simulink model "lc_filt_2"  (Simulink 7.4)
settings: Solver=ode45  StartTime=0.0  StopTime=10.0  MaxStep=1/(5*5e6)  RelTol=1e-3
InitFcn:
  | [l,c]=qsynth('getLC')
values from neighbouring files (symbols this model uses):
  a = [1 5726176.52661 1.28574552517e+14 5.97941269361e+20 5.92183808786e+27 2.12384980348e+34 1.13676377206e+41 2.81047410932e+47 7.39377027116e+53 8.72797204109e+59]    [lpf_coefs.mat]    (also in qsynth.m = 1)
  b = [0 36915.6508509 -1.25549596846e-06 1.20108825102e+19 -347373112.51 1.28132141519e+33 -2.666806229e+22 5.6099849733e+46 -6.09794797058e+35 8.72797204109e+59]    [lpf_coefs.mat]    (also in qsynth.m = 0)
  c = [1.7464e-07 0 2.8303e-07 0 2.0989e-07 0 1.304e-07 0 4.9154e-08]    [lcvalues.mat]    (also in qsynth.m = 1/val1)
  d = 1    [qsynth.m]
  l = [0 2.1751e-07 2.1186e-08 2.0002e-07 7.2973e-08 1.4884e-07 1.5754e-07 1.3878e-07 4.5617e-07]    [lcvalues.mat]
undefined symbols (not defined in the file or in its folder): Fs, magnitude
libraries: powerlib x14, dspindex x6, dspsigops x3, dspbuff3 x2, dspxfrm3 x2, dsparch3 x2, dspsnks4 x2, dspmtrx3 x1, simulink x1
settings Model: Creator=Owner  LastModifiedBy=Dick
settings DataIOCC: SignalLoggingName=sigsOut
settings OptimizationCC: BooleanDataType=off  InlineInvariantSignals=on  InitFltsAndDblsToZero=on
settings DebuggingCC: SaveWithParameterizedLinksMsg=none  SignalResolutionControl=TryResolveAllWithWarning  SolverPrmCheckMsg=none  MultiTaskDSMMsg=warning  MultiTaskCondExecSysMsg=none  StrictBusMsg=None
settings HardwareCC: TargetUnknown=on
settings RTWCC: IncludeERTFirstTime=on
settings GRTTargetCC: TargetFcnLib=ansi_tfl_tmw.mat

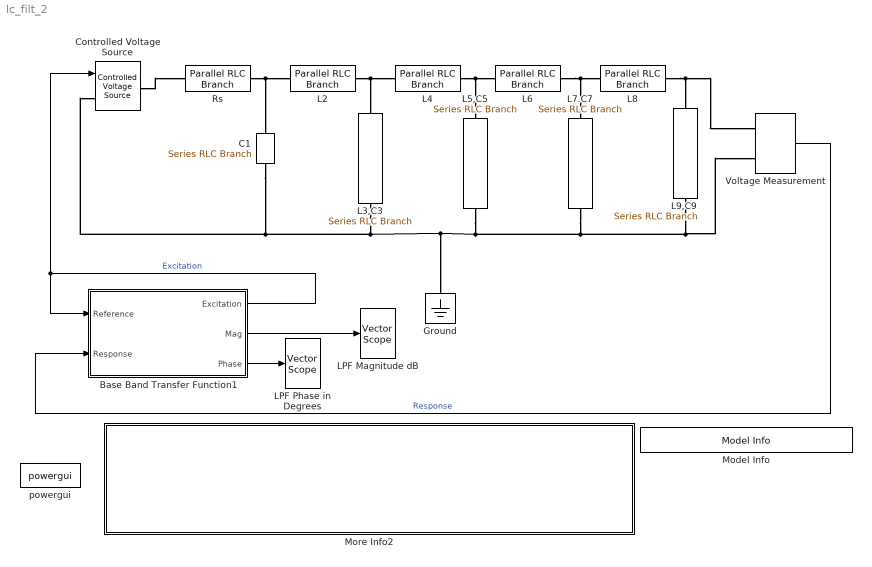
== system lc_filt_2 ==
  " L2" : powerlib/Elements/Parallel RLC Branch  DialogController=POWERSYS.PowerSysDialog  PhysicalDomain=powersysdomain  SubClassName=unknown  LeftPortType=p1  RightPortType=p1  LConnTagsString=a  RConnTagsString=__new0  BranchType=L  Resistance=1.0  Inductance=l(2)  SetiL0=off  InitialCurrent=0  Capacitance=1.0  Setx0=off  InitialVoltage=0  Measurements=None
  " L4" : powerlib/Elements/Parallel RLC Branch  DialogController=POWERSYS.PowerSysDialog  PhysicalDomain=powersysdomain  SubClassName=unknown  LeftPortType=p1  RightPortType=p1  LConnTagsString=a  RConnTagsString=__new0  BranchType=L  Resistance=1.0  Inductance=l(4)  SetiL0=off  InitialCurrent=0  Capacitance=1.0  Setx0=off  InitialVoltage=0  Measurements=None
  " L6" : powerlib/Elements/Parallel RLC Branch  DialogController=POWERSYS.PowerSysDialog  PhysicalDomain=powersysdomain  SubClassName=unknown  LeftPortType=p1  RightPortType=p1  LConnTagsString=a  RConnTagsString=__new0  BranchType=L  Resistance=1.0  Inductance=l(6)  SetiL0=off  InitialCurrent=0  Capacitance=1.0  Setx0=off  InitialVoltage=0  Measurements=None
  " L8" : powerlib/Elements/Parallel RLC Branch  DialogController=POWERSYS.PowerSysDialog  PhysicalDomain=powersysdomain  SubClassName=unknown  LeftPortType=p1  RightPortType=p1  LConnTagsString=a  RConnTagsString=__new0  BranchType=L  Resistance=1.0  Inductance=l(8)  SetiL0=off  InitialCurrent=0  Capacitance=1.0  Setx0=off  InitialVoltage=0  Measurements=None
  " Rs" : powerlib/Elements/Parallel RLC Branch  DialogController=POWERSYS.PowerSysDialog  PhysicalDomain=powersysdomain  SubClassName=unknown  LeftPortType=p1  RightPortType=p1  LConnTagsString=a  RConnTagsString=__new0  BranchType=R  Resistance=1  Inductance=1.0  SetiL0=off  InitialCurrent=0  Capacitance=1.0  Setx0=off  InitialVoltage=0  Measurements=None
  Base Band Transfer Function1 : Subsystem  Description=Spectrum Analyzer  mask{BW=5e6, NFFT=1024, Avg_fac=100}
      mask prompts: BW "Bandwidth"; NFFT "FFT Length (power of 2)"; Avg_fac "Averaging Factor (>=1)"
  C1 : powerlib/Elements/Series RLC Branch  DialogController=POWERSYS.PowerSysDialog  PhysicalDomain=powersysdomain  SubClassName=unknown  LeftPortType=p1  RightPortType=p1  LConnTagsString=__new0  RConnTagsString=__new0  BranchType=C  Resistance=1.0  Inductance=1.0  SetiL0=off  InitialCurrent=0  Capacitance=c(1)  Setx0=off  InitialVoltage=0  Measurements=None
  Controlled Voltage Source : powerlib/Electrical Sources/Controlled Voltage Source  DialogController=POWERSYS.PowerSysDialog  SystemSampleTime=-1  Initialize=off  Source_Type=AC  Amplitude=100  Phase=0  Frequency=0  Measurements=Voltage
  Ground : powerlib/Elements/Ground  DialogController=POWERSYS.PowerSysDialog  PhysicalDomain=powersysdomain  SubClassName=unknown  LeftPortType=p1  RightPortType=p1  LConnTagsString=a
  L3,C3 : powerlib/Elements/Series RLC Branch  DialogController=POWERSYS.PowerSysDialog  PhysicalDomain=powersysdomain  SubClassName=unknown  LeftPortType=p1  RightPortType=p1  LConnTagsString=__new0  RConnTagsString=__new0  BranchType=LC  Resistance=1.0  Inductance=l(3)  SetiL0=off  InitialCurrent=0  Capacitance=c(3)  Setx0=off  InitialVoltage=0  Measurements=None
  L5,C5 : powerlib/Elements/Series RLC Branch  DialogController=POWERSYS.PowerSysDialog  PhysicalDomain=powersysdomain  SubClassName=unknown  LeftPortType=p1  RightPortType=p1  LConnTagsString=__new0  RConnTagsString=__new0  BranchType=LC  Resistance=1.0  Inductance=l(5)  SetiL0=off  InitialCurrent=0  Capacitance=c(5)  Setx0=off  InitialVoltage=0  Measurements=None
  L7.C7 : powerlib/Elements/Series RLC Branch  DialogController=POWERSYS.PowerSysDialog  PhysicalDomain=powersysdomain  SubClassName=unknown  LeftPortType=p1  RightPortType=p1  LConnTagsString=__new0  RConnTagsString=__new0  BranchType=LC  Resistance=1.0  Inductance=l(7)  SetiL0=off  InitialCurrent=0  Capacitance=c(7)  Setx0=off  InitialVoltage=0  Measurements=None
  "L9,C9 " : powerlib/Elements/Series RLC Branch  DialogController=POWERSYS.PowerSysDialog  PhysicalDomain=powersysdomain  SubClassName=unknown  LeftPortType=p1  RightPortType=p1  LConnTagsString=__new0  RConnTagsString=__new0  BranchType=LC  Resistance=1.0  Inductance=l(9)  SetiL0=off  InitialCurrent=0  Capacitance=c(9)  Setx0=off  InitialVoltage=0  Measurements=None
  LPF Magnitude dB : dspsnks4/Vector Scope  DialogController=dspdialog.VectorScope  DialogControllerArgs=DataTag5  ScopeProperties=on  Domain=Frequency  HorizSpan=1  DisplayProperties=off  AxisGrid=on  Memory=off  FrameNumber=on  AxisLegend=off  AxisZoom=off  OpenScopeAtSimStart=on  OpenScopeImmediately=off  FigPos=[15 321 372 236]  AxisProperties=off  XUnits=Hertz  XRange=[0...Fs/2]  InheritXIncr=on  XIncr=2*Fs  XLabel=Time  XLimit=Auto  XMin=0  XMax=1  XStart=0  YUnits=dB  YLabel=dB  LineProperties=off  LineColors=[1 0 0]|[1 0 0]  XAxisParamsVer=6.8
      settings: YMin=-100  YMax=10
  LPF Phase in Degrees : dspsnks4/Vector Scope  DialogController=dspdialog.VectorScope  DialogControllerArgs=DataTag6  ScopeProperties=on  Domain=Frequency  HorizSpan=1  DisplayProperties=off  AxisGrid=on  Memory=off  FrameNumber=on  AxisLegend=off  AxisZoom=off  OpenScopeAtSimStart=on  OpenScopeImmediately=off  FigPos=[16 37 372 236]  AxisProperties=off  XUnits=Hertz  XRange=[0...Fs/2]  InheritXIncr=on  XIncr=1  XLabel=Frequency  XLimit=Auto  XMin=0  XMax=1  XStart=0  YUnits=Magnitude  YLabel=Phase in Degrees  LineProperties=off  LineColors=[1 0 0]  XAxisParamsVer=6.8
      settings: YMin=-892.290290597093  YMax=45.3005092441757
  Model Info : simulink/Model-Wide Utilities/Model Info  SystemSampleTime=-1  InitialBlockCM=None  BlockCM=None  Frame=on  DisplayStringWithTags=Copywrite 2005-2010 The MathWorks, Inc.  HorizontalTextAlignment=Center  LeftAlignmentValue=0.5  SourceBlockDiagram=lc_filt_2  TagMaxNumber=20
  More Info2 : Subsystem
      settings: OpenFcn=qsynth
      mask Display: disp('1) Double click here to synthesize LC filter. Use N=9, Rs=1 Rl=inf Fc=1e6 \n 2) Synthesize the filter, do not close GUI,  then return to this model and start the simulation. \n 3) The LC filter is "measured" with the Base Band Transfer Function Estimator \n ')
  Voltage Measurement : powerlib/Measurements/Voltage Measurement  DialogController=POWERSYS.PowerSysDialog  SystemSampleTime=-1  PhasorSimulation=off  OutputType=Magnitude  PSBequivalent=0
  powergui : powerlib/powergui  SystemSampleTime=-1  SimulationMode=Continuous  SampleTime=0  frequency=60  SPID=off  DisableSnubberDevices=off  DisableRonSwitches=off  DisableVfSwitches=off  SwTol=0  Interpol=off  frequencyindice=0  echomessages=off  HookPort=off  DisplayEquations=off  FunctionMessages=off  EnableUseOfTLC=off  x0status=blocks  RestoreLinks=warning  Frange=[0:2:500]  Ylog=off  Xlog=on  ShowGrid=off  save=off  variable=ZData  ZoomFFT=on  StartTime=0.0  cycles=1  DisplayStyle=1  fundamental=60  FreqAxis=off  MaxFrequency=1000  frequencyindicesteady=1  RmsSteady=1  display=off  Ts=0  methode=off
  wires:
  Voltage Measurement/1 -> Base Band Transfer Function1/2(Response)  "Response"
  Base Band Transfer Function1/2(Mag) -> LPF Magnitude dB/1
  Base Band Transfer Function1/3(Phase) -> LPF Phase in Degrees/1
  Base Band Transfer Function1/1(Excitation) -> Controlled Voltage Source/1, Base Band Transfer Function1/1("Reference ")  "Excitation"
  connections:
  " Rs"/RConn1 -- C1/LConn1 -- " L2"/LConn1
  " L2"/RConn1 -- L3,C3/LConn1 -- " L4"/LConn1
  " L4"/RConn1 -- L5,C5/LConn1 -- " L6"/LConn1
  " L6"/RConn1 -- L7.C7/LConn1 -- " L8"/LConn1
  L5,C5/RConn1 -- L7.C7/RConn1 -- "L9,C9 "/RConn1 -- Voltage Measurement/LConn2 -- L3,C3/RConn1 -- C1/RConn1 -- Controlled Voltage Source/LConn1 -- Ground/LConn1
  Controlled Voltage Source/RConn1 -- " Rs"/LConn1
  " L8"/RConn1 -- Voltage Measurement/LConn1 -- "L9,C9 "/LConn1

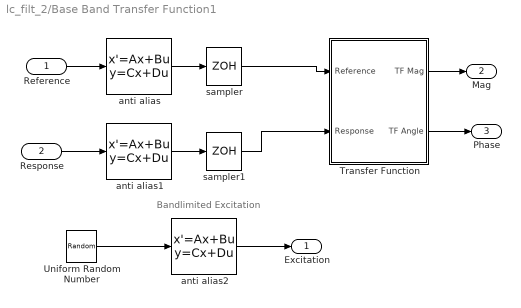
== system lc_filt_2/Base Band Transfer Function1 ==
  note: Bandlimited Excitation
  "Reference " : Inport  OutDataType=sfix(16)  OutScaling=2^0
  Response : Inport  Port=2  OutDataType=sfix(16)  OutScaling=2^0
  "Transfer Function " : Subsystem  mask{NFFT=NFFT, Navg=Avg_fac, pcnt=100/1.28, unwrap_flag=on}
      mask prompts: NFFT "FFT length (power of 2):"; Navg "Spectral Averaging Factor (>=1):"; pcnt "Percentage of  Alias Free Data  (<=100)"; unwrap_flag "Unwrap Phase"
      mask Display: disp('Transfer Function \n Estimation (v2.0) ')
  Uniform Random Number : UniformRandomNumber  SampleTime=1/(2.56*BW)
  anti alias : StateSpace  AncestorBlock=dsparch3/Analog Filter Design  A=a  B=b  C=c  D=d  mask(Analog Filter Design){method=Elliptic, filttype=Lowpass, N=8, Wlo=BW*2*pi, Whi=80, Rp=2, Rs=100}
      mask prompts: method "Design method:"; filttype "Filter type:"; N "Filter order:"; Wlo "Passband edge frequency (rad/s):"; Whi "(unused)"; Rp "Passband ripple in dB:"; Rs "Stopband attenuation in dB:"
      mask help: Design one of several standard analog filters, implemented in state-space form.
      mask init:
      | [a,b,c,d,h,w,str]=dspblkanalog('design', method,filttype,N,Wlo,Whi,Rp,Rs);
      mask Help: web(dspbhelp);
      mask StyleString: popup(Butterworth|Chebyshev I|Chebyshev II|Elliptic|Bessel),popup(Lowpass|Highpass|Bandpass|Bandstop),edit,edit,edit,edit,edit
      mask CallbackString: dspblkanalog|dspblkanalog|||||
      mask Display: plot(w,h); text(.05,.9,str);
  anti alias1 : StateSpace  AncestorBlock=dsparch3/Analog Filter Design  A=a  B=b  C=c  D=d  mask(Analog Filter Design){method=Elliptic, filttype=Lowpass, N=8, Wlo=BW*2*pi, Whi=80, Rp=2, Rs=100}
      mask prompts: method "Design method:"; filttype "Filter type:"; N "Filter order:"; Wlo "Passband edge frequency (rad/s):"; Whi "(unused)"; Rp "Passband ripple in dB:"; Rs "Stopband attenuation in dB:"
      mask help: Design one of several standard analog filters, implemented in state-space form.
      mask init:
      | [a,b,c,d,h,w,str]=dspblkanalog('design', method,filttype,N,Wlo,Whi,Rp,Rs);
      mask Help: web(dspbhelp);
      mask StyleString: popup(Butterworth|Chebyshev I|Chebyshev II|Elliptic|Bessel),popup(Lowpass|Highpass|Bandpass|Bandstop),edit,edit,edit,edit,edit
      mask CallbackString: dspblkanalog|dspblkanalog|||||
      mask Display: plot(w,h); text(.05,.9,str);
  anti alias2 : StateSpace  AncestorBlock=dsparch3/Analog Filter Design  A=a  B=b  C=c  D=d  mask(Analog Filter Design){method=Elliptic, filttype=Lowpass, N=8, Wlo=BW*2*pi, Whi=80, Rp=2, Rs=100}
      mask prompts: method "Design method:"; filttype "Filter type:"; N "Filter order:"; Wlo "Passband edge frequency (rad/s):"; Whi "(unused)"; Rp "Passband ripple in dB:"; Rs "Stopband attenuation in dB:"
      mask help: Design one of several standard analog filters, implemented in state-space form.
      mask init:
      | [a,b,c,d,h,w,str]=dspblkanalog('design', method,filttype,N,Wlo,Whi,Rp,Rs);
      mask Help: web(dspbhelp);
      mask StyleString: popup(Butterworth|Chebyshev I|Chebyshev II|Elliptic|Bessel),popup(Lowpass|Highpass|Bandpass|Bandstop),edit,edit,edit,edit,edit
      mask CallbackString: dspblkanalog|dspblkanalog|||||
      mask Display: plot(w,h); text(.05,.9,str);
  sampler : ZeroOrderHold  SampleTime=1/(2.56*BW)
  sampler1 : ZeroOrderHold  SampleTime=1/(2.56*BW)
  Excitation : Outport  OutDataType=sfix(16)  OutScaling=2^0
  Mag : Outport  Port=2  OutDataType=sfix(16)  OutScaling=2^0
  Phase : Outport  Port=3  OutDataType=sfix(16)  OutScaling=2^0
  wires:
  "Transfer Function "/2(TF Angle) -> Phase/1
  "Transfer Function "/1(TF Mag) -> Mag/1
  sampler1/1 -> "Transfer Function "/2(Response)
  sampler/1 -> "Transfer Function "/1(Reference)
  anti alias2/1 -> Excitation/1
  Uniform Random Number/1 -> anti alias2/1
  Response/1 -> anti alias1/1
  anti alias1/1 -> sampler1/1
  "Reference "/1 -> anti alias/1
  anti alias/1 -> sampler/1

== system lc_filt_2/More Info2 ==

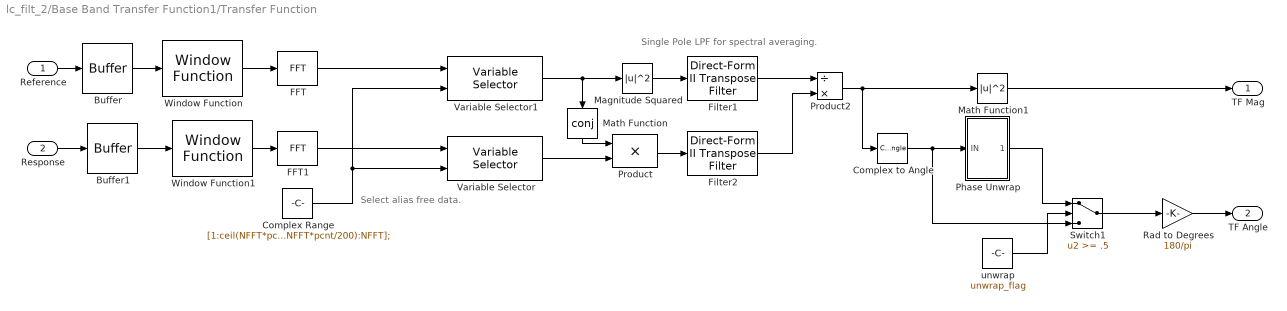
== system lc_filt_2/Base Band Transfer Function1/Transfer Function  ==
  note: Single Pole LPF for spectral averaging.
  note: Select alias free data.
  Reference : Inport  OutDataType=sfix(16)  OutScaling=2^0
  Response : Inport  Port=2  OutDataType=sfix(16)  OutScaling=2^0
  Buffer : dspbuff3/Buffer  N=NFFT  V=0  ic=0
  Buffer1 : dspbuff3/Buffer  N=NFFT  V=0  ic=0
  Complex Range : Constant  Value=[1:ceil(NFFT*pcnt/200),ceil(1+NFFT-NFFT*pcnt/200):NFFT];  OutDataType=sfix(16)  OutScaling=2^0
  Complex to Angle : ComplexToMagnitudeAngle  Output=Angle
  FFT : dspxfrm3/FFT  DialogController=dspDDGCreate  DialogControllerArgs=DataTag0  CompMethod=Table lookup  TableOpt=Speed  BitRevOrder=off  InheritFFTLength=on  FFTLength=64  SkipNorm=off  firstCoeffMode=Specify word length  firstCoeffWordLength=16  firstCoeffFracLength=15  roundingMode=Floor  overflowMode=off
  FFT1 : dspxfrm3/FFT  DialogController=dspDDGCreate  DialogControllerArgs=DataTag1  CompMethod=Table lookup  TableOpt=Speed  BitRevOrder=off  InheritFFTLength=on  FFTLength=64  SkipNorm=off  firstCoeffMode=User-defined  firstCoeffWordLength=16  firstCoeffFracLength=15  roundingMode=Floor  overflowMode=off
  Filter1 : dsparch3/Direct-Form II Transpose Filter  num=1  den=[Navg -(Navg-1)]  ic=eps
  Filter2 : dsparch3/Direct-Form II Transpose Filter  num=1  den=[Navg -(Navg-1)]  ic=eps
  Magnitude Squared : Math  Operator=magnitude^2  OutDataType=sfix(16)  OutScaling=2^0  SaturateOnIntegerOverflow=on
  Math Function : Math  Operator=conj  OutDataType=sfix(16)  OutScaling=2^0  SaturateOnIntegerOverflow=on
  Math Function1 : Math  Operator=magnitude^2  OutDataType=sfix(16)  OutScaling=2^0  SaturateOnIntegerOverflow=on
  Phase Unwrap : Subsystem
  Product : Product  OutDataType=sfix(16)  OutScaling=2^0  SaturateOnIntegerOverflow=on  InputSameDT=on  OutDataTypeStr=Inherit: Same as first input
  Product2 : Product  Inputs=/*  OutDataType=sfix(16)  OutScaling=2^0  SaturateOnIntegerOverflow=on  InputSameDT=on  OutDataTypeStr=Inherit: Same as first input
  Rad to Degrees : Gain  Gain=180/pi  ParameterDataType=sfix(16)  ParameterScaling=2^0  OutDataType=sfix(16)  OutScaling=2^0
  Switch1 : Switch  Threshold=.5
  Variable Selector : dspindex/Variable Selector  NumInputs=1  rowsOrCols=Rows  IdxMode=Variable  Elements=[1 3]  ZerOneIdxMode=One-based  errmode=Clip Index  FillMode=on  FillValues=0
  Variable Selector1 : dspindex/Variable Selector  NumInputs=1  rowsOrCols=Rows  IdxMode=Variable  Elements=[1 3]  ZerOneIdxMode=One-based  errmode=Clip Index  FillMode=on  FillValues=0
  Window Function : dspsigops/Window Function  DialogController=dspDDGCreate  DialogControllerArgs=DataTag3  winmode=Apply window to input  wintype=Hann  sampmode=Continuous  samptime=1  N=64  Rs=50  beta=10  winsamp=Periodic  UserWindow=hamming  OptParams=off  UserParams={'symmetric'}  dataType=double  isSigned=on  wordLen=16  udDataType=sfix(16)  fracBitsMode=Best precision  numFracBits=15  roundingMode=Floor  overflowMode=off  numSidelobes=4  sidelobeLevel=-30
  Window Function1 : dspsigops/Window Function  DialogController=dspDDGCreate  DialogControllerArgs=DataTag4  winmode=Apply window to input  wintype=Hann  sampmode=Continuous  samptime=1  N=64  Rs=50  beta=10  winsamp=Periodic  UserWindow=hamming  OptParams=off  UserParams={'symmetric'}  dataType=double  isSigned=on  wordLen=16  udDataType=sfix(16)  fracBitsMode=Best precision  numFracBits=15  roundingMode=Floor  overflowMode=off  numSidelobes=4  sidelobeLevel=-30
  unwrap : Constant  Value=unwrap_flag  OutDataType=sfix(16)  OutScaling=2^0
  TF Mag : Outport  OutDataType=sfix(16)  OutScaling=2^0
  TF Angle : Outport  Port=2  OutDataType=sfix(16)  OutScaling=2^0
  wires:
  Complex Range/1 -> Variable Selector/2, Variable Selector1/2
  Complex to Angle/1 -> Switch1/3, Phase Unwrap/1(IN)
  Rad to Degrees/1 -> TF Angle/1
  Response/1 -> Buffer1/1
  Reference/1 -> Buffer/1
  Product/1 -> Filter2/1
  FFT1/1 -> Variable Selector/1
  Math Function/1 -> Product/1
  Magnitude Squared/1 -> Filter1/1
  FFT/1 -> Variable Selector1/1
  Math Function1/1 -> TF Mag/1
  Window Function/1 -> FFT/1
  Window Function1/1 -> FFT1/1
  Filter1/1 -> Product2/1
  Filter2/1 -> Product2/2
  Buffer/1 -> Window Function/1
  Buffer1/1 -> Window Function1/1
  Product2/1 -> Complex to Angle/1, Math Function1/1
  Variable Selector/1 -> Product/2
  Variable Selector1/1 -> Magnitude Squared/1, Math Function/1
  Switch1/1 -> Rad to Degrees/1
  unwrap/1 -> Switch1/2
  Phase Unwrap/1(Out1) -> Switch1/1

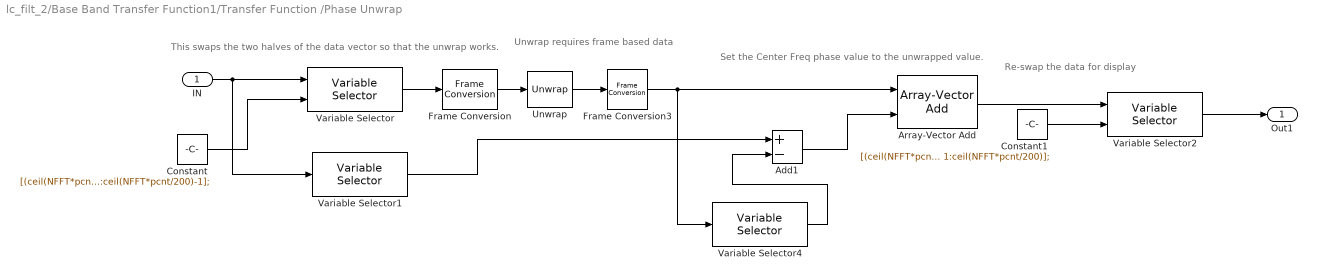
== system lc_filt_2/Base Band Transfer Function1/Transfer Function /Phase Unwrap ==
  note: This swaps the two halves of the data vector
      | so that the unwrap works.
  note: Set the Center Freq phase value to the unwrapped value.
  note: Re-swap the data for display
  note: Unwrap requires frame based data
  IN : Inport  OutDataType=sfix(16)  OutScaling=2^0
  Add1 : Sum  Inputs=+-  OutDataType=sfix(16)  OutScaling=2^-10
  Array-Vector Add : dspmtrx3/Array-Vector Add  DialogController=dspDDGCreate  DialogControllerArgs=DataTag2  Dimension=2  V_Source=Input port  V_VectFromMask=[0.5 0.25]  roundingMode=Floor  overflowMode=off
  Constant : Constant  Value=[(ceil(NFFT*pcnt/200)):ceil(NFFT*pcnt/100) 1:ceil(NFFT*pcnt/200)-1];  OutDataType=sfix(16)  OutScaling=2^0
  Constant1 : Constant  Value=[(ceil(NFFT*pcnt/200)+1):ceil(NFFT*pcnt/100) 1:ceil(NFFT*pcnt/200)];  OutDataType=sfix(16)  OutScaling=2^0
  Frame Conversion : FrameConversion
  Frame Conversion3 : FrameConversion  OutFrame=Sample-based
  Unwrap : dspsigops/Unwrap  running=on  tol=pi
  Variable Selector : dspindex/Variable Selector  NumInputs=1  rowsOrCols=Rows  IdxMode=Variable  Elements=[1 3]  ZerOneIdxMode=One-based  errmode=Clip Index  FillMode=on  FillValues=0
  Variable Selector1 : dspindex/Variable Selector  NumInputs=1  rowsOrCols=Rows  IdxMode=Fixed  Elements=[1]  ZerOneIdxMode=One-based  errmode=Clip Index  FillMode=on  FillValues=0
  Variable Selector2 : dspindex/Variable Selector  NumInputs=1  rowsOrCols=Rows  IdxMode=Variable  Elements=[1 3]  ZerOneIdxMode=One-based  errmode=Clip Index  FillMode=on  FillValues=0
  Variable Selector4 : dspindex/Variable Selector  NumInputs=1  rowsOrCols=Rows  IdxMode=Fixed  Elements=length([(ceil(NFFT*pcnt/200)+1):ceil(NFFT*pcnt/100) 1:ceil(NFFT*pcnt/200)] )/2+1  ZerOneIdxMode=One-based  errmode=Clip Index  FillMode=on  FillValues=0
  Out1 : Outport  OutDataType=sfix(16)  OutScaling=2^0
  wires:
  Frame Conversion/1 -> Unwrap/1
  Variable Selector2/1 -> Out1/1
  IN/1 -> Variable Selector/1, Variable Selector1/1
  Constant/1 -> Variable Selector/2
  Variable Selector/1 -> Frame Conversion/1
  Variable Selector1/1 -> Add1/1
  Unwrap/1 -> Frame Conversion3/1
  Variable Selector4/1 -> Add1/2
  Constant1/1 -> Variable Selector2/2
  Frame Conversion3/1 -> Variable Selector4/1, Array-Vector Add/1
  Add1/1 -> Array-Vector Add/2
  Array-Vector Add/1 -> Variable Selector2/1
